simulink model "TST_CoETM_ClgDem"  (R2016b)
settings: Solver=FixedStepDiscrete  StartTime=0.0  StopTime=simTime  FixedStep=sampleTime  RelTol=1e-3
values from neighbouring files (symbols this model uses):
  testCase = 1    [initTST_CoETM_ClgDem_001.m]    (also in initTST_CoETM_ClgDem_002.m = 2)
libraries: simulink x7, UnitTest_Lib x4
settings Model: Creator=xinchangran  LastModifiedBy=xinchangran
settings DebuggingCC: SignalRangeChecking=error

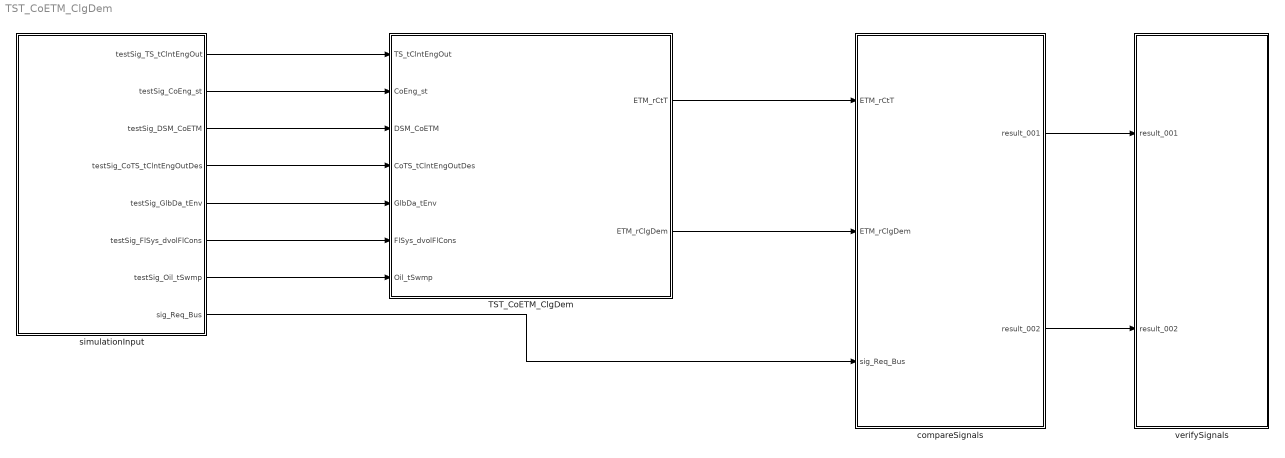
== system TST_CoETM_ClgDem ==
  TST_CoETM_ClgDem : Subsystem
  compareSignals : Subsystem
  simulationInput : Subsystem
  verifySignals : Subsystem
  wires:
  simulationInput/1(testSig_TS_tClntEngOut) -> TST_CoETM_ClgDem/1(TS_tClntEngOut)
  simulationInput/2(testSig_CoEng_st) -> TST_CoETM_ClgDem/2(CoEng_st)
  simulationInput/3(testSig_DSM_CoETM) -> TST_CoETM_ClgDem/3(DSM_CoETM)
  simulationInput/4(testSig_CoTS_tClntEngOutDes) -> TST_CoETM_ClgDem/4(CoTS_tClntEngOutDes)
  simulationInput/5(testSig_GlbDa_tEnv) -> TST_CoETM_ClgDem/5(GlbDa_tEnv)
  simulationInput/6(testSig_FlSys_dvolFlCons) -> TST_CoETM_ClgDem/6(FlSys_dvolFlCons)
  simulationInput/7(testSig_Oil_tSwmp) -> TST_CoETM_ClgDem/7(Oil_tSwmp)
  TST_CoETM_ClgDem/1(ETM_rCtT) -> compareSignals/1(ETM_rCtT)
  TST_CoETM_ClgDem/2(ETM_rClgDem) -> compareSignals/2(ETM_rClgDem)
  simulationInput/8(sig_Req_Bus) -> compareSignals/3(sig_Req_Bus)
  compareSignals/1(result_001) -> verifySignals/1(result_001)
  compareSignals/2(result_002) -> verifySignals/2(result_002)

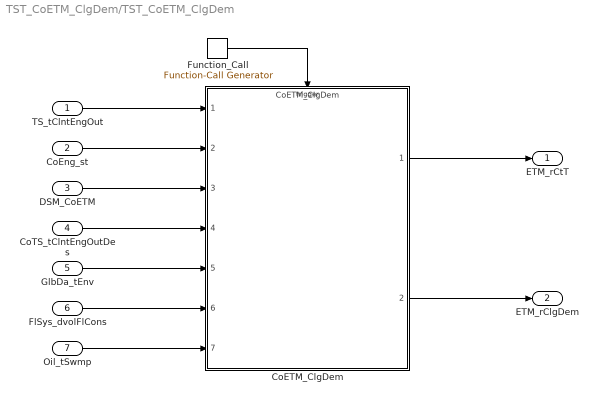
== system TST_CoETM_ClgDem/TST_CoETM_ClgDem ==
  TS_tClntEngOut : Inport
  CoEng_st : Inport  Port=2
  DSM_CoETM : Inport  Port=3
  CoTS_tClntEngOutDes : Inport  Port=4
  GlbDa_tEnv : Inport  Port=5
  FlSys_dvolFlCons : Inport  Port=6
  Oil_tSwmp : Inport  Port=7
  CoETM_ClgDem : ModelReference  ModelNameDialog=CoETM_ClgDem  SimulationMode=Normal  ModelReferenceVersion=1.155  TriggerPortName=function  TriggerPortTriggerType=function-call  TriggerPortStatesWhenEnabling=held
  Function_Call : simulink/Ports & Subsystems/Function-Call Generator  sample_time=sampleTime  numberOfIterations=1
  ETM_rCtT : Outport
  ETM_rClgDem : Outport  Port=2
  wires:
  Function_Call/1 -> CoETM_ClgDem/Trigger
  TS_tClntEngOut/1 -> CoETM_ClgDem/1
  CoEng_st/1 -> CoETM_ClgDem/2
  DSM_CoETM/1 -> CoETM_ClgDem/3
  CoTS_tClntEngOutDes/1 -> CoETM_ClgDem/4
  GlbDa_tEnv/1 -> CoETM_ClgDem/5
  FlSys_dvolFlCons/1 -> CoETM_ClgDem/6
  Oil_tSwmp/1 -> CoETM_ClgDem/7
  CoETM_ClgDem/1 -> ETM_rCtT/1
  CoETM_ClgDem/2 -> ETM_rClgDem/1

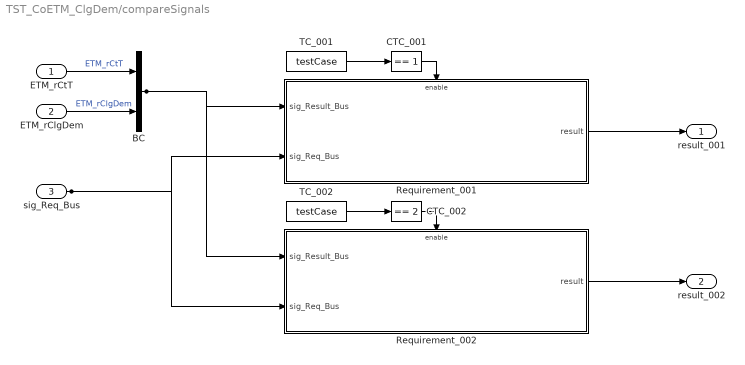
== system TST_CoETM_ClgDem/compareSignals ==
  ETM_rCtT : Inport
  ETM_rClgDem : Inport  Port=2
  sig_Req_Bus : Inport  Port=3
  BC : BusCreator  Inputs=2
  CTC_001 : simulink/Logic and Bit Operations/Compare To Constant  relop===  const=1  OutDataTypeStr=boolean
  CTC_002 : simulink/Logic and Bit Operations/Compare To Constant  relop===  const=2  OutDataTypeStr=boolean
  Requirement_001 : Subsystem
  Requirement_002 : Subsystem
  TC_001 : Constant  Value=testCase
  TC_002 : Constant  Value=testCase
  result_001 : Outport
  result_002 : Outport  Port=2
  wires:
  ETM_rCtT/1 -> BC/1  "ETM_rCtT"
  ETM_rClgDem/1 -> BC/2  "ETM_rClgDem"
  TC_001/1 -> CTC_001/1
  CTC_001/1 -> Requirement_001/Enable
  sig_Req_Bus/1 -> Requirement_001/2(sig_Req_Bus), Requirement_002/2(sig_Req_Bus)
  BC/1 -> Requirement_001/1(sig_Result_Bus), Requirement_002/1(sig_Result_Bus)
  Requirement_001/1(result) -> result_001/1
  TC_002/1 -> CTC_002/1
  CTC_002/1 -> Requirement_002/Enable
  Requirement_002/1(result) -> result_002/1

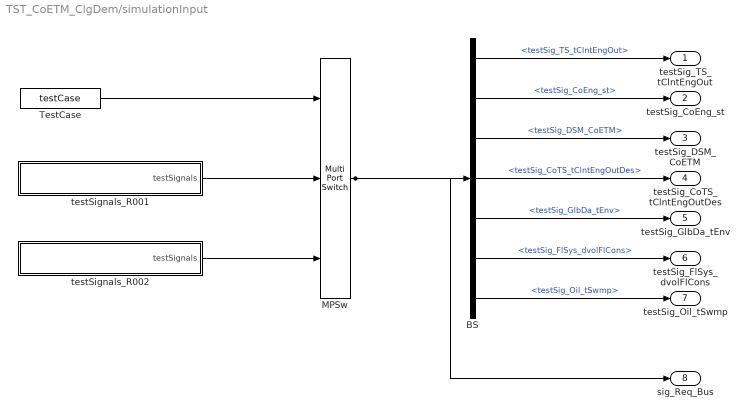
== system TST_CoETM_ClgDem/simulationInput ==
  BS : BusSelector  OutputSignals=testSig_TS_tClntEngOut,testSig_CoEng_st,testSig_DSM_CoETM,testSig_CoTS_tClntEngOutDes,testSig_GlbDa_tEnv,testSig_FlSys_dvolFlCons,testSig_Oil_tSwmp
  MPSw : MultiPortSwitch  Inputs=2  SaturateOnIntegerOverflow=on  InputSameDT=on
  TestCase : Constant  Value=testCase
  testSignals_R001 : Subsystem
  testSignals_R002 : Subsystem
  testSig_TS_tClntEngOut : Outport
  testSig_CoEng_st : Outport  Port=2
  testSig_DSM_CoETM : Outport  Port=3
  testSig_CoTS_tClntEngOutDes : Outport  Port=4
  testSig_GlbDa_tEnv : Outport  Port=5
  testSig_FlSys_dvolFlCons : Outport  Port=6
  testSig_Oil_tSwmp : Outport  Port=7
  sig_Req_Bus : Outport  Port=8
  wires:
  BS/1 -> testSig_TS_tClntEngOut/1  "<testSig_TS_tClntEngOut>"
  BS/2 -> testSig_CoEng_st/1  "<testSig_CoEng_st>"
  BS/3 -> testSig_DSM_CoETM/1  "<testSig_DSM_CoETM>"
  BS/4 -> testSig_CoTS_tClntEngOutDes/1  "<testSig_CoTS_tClntEngOutDes>"
  BS/5 -> testSig_GlbDa_tEnv/1  "<testSig_GlbDa_tEnv>"
  BS/6 -> testSig_FlSys_dvolFlCons/1  "<testSig_FlSys_dvolFlCons>"
  BS/7 -> testSig_Oil_tSwmp/1  "<testSig_Oil_tSwmp>"
  MPSw/1 -> BS/1, sig_Req_Bus/1
  TestCase/1 -> MPSw/1
  testSignals_R001/1(testSignals) -> MPSw/2
  testSignals_R002/1(testSignals) -> MPSw/3

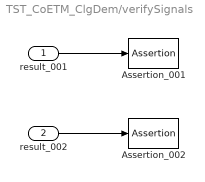
== system TST_CoETM_ClgDem/verifySignals ==
  result_001 : Inport
  result_002 : Inport  Port=2
  Assertion_001 : Assertion  Enabled=off
  Assertion_002 : Assertion  Enabled=off
  wires:
  result_001/1 -> Assertion_001/1
  result_002/1 -> Assertion_002/1

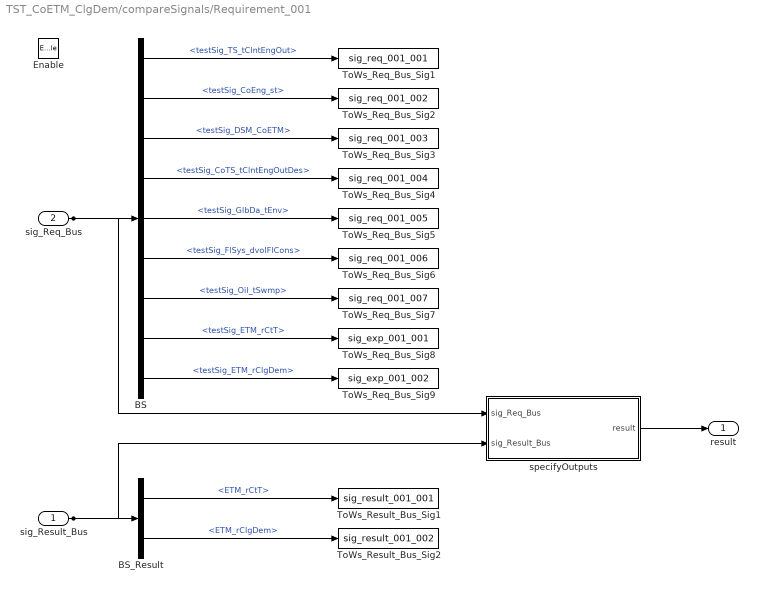
== system TST_CoETM_ClgDem/compareSignals/Requirement_001 ==
  sig_Result_Bus : Inport
  sig_Req_Bus : Inport  Port=2
  Enable : EnablePort
  BS : BusSelector  OutputSignals=testSig_TS_tClntEngOut,testSig_CoEng_st,testSig_DSM_CoETM,testSig_CoTS_tClntEngOutDes,testSig_GlbDa_tEnv,testSig_FlSys_dvolFlCons,testSig_Oil_tSwmp,testSig_ETM_rCtT,testSig_ETM_rClgDem
  BS_Result : BusSelector  OutputSignals=ETM_rCtT,ETM_rClgDem
  ToWs_Req_Bus_Sig1 : ToWorkspace  VariableName=sig_req_001_001  SaveFormat=Structure With Time
  ToWs_Req_Bus_Sig2 : ToWorkspace  VariableName=sig_req_001_002  SaveFormat=Structure With Time
  ToWs_Req_Bus_Sig3 : ToWorkspace  VariableName=sig_req_001_003  SaveFormat=Structure With Time
  ToWs_Req_Bus_Sig4 : ToWorkspace  VariableName=sig_req_001_004  SaveFormat=Structure With Time
  ToWs_Req_Bus_Sig5 : ToWorkspace  VariableName=sig_req_001_005  SaveFormat=Structure With Time
  ToWs_Req_Bus_Sig6 : ToWorkspace  VariableName=sig_req_001_006  SaveFormat=Structure With Time
  ToWs_Req_Bus_Sig7 : ToWorkspace  VariableName=sig_req_001_007  SaveFormat=Structure With Time
  ToWs_Req_Bus_Sig8 : ToWorkspace  VariableName=sig_exp_001_001  SaveFormat=Structure With Time
  ToWs_Req_Bus_Sig9 : ToWorkspace  VariableName=sig_exp_001_002  SaveFormat=Structure With Time
  ToWs_Result_Bus_Sig1 : ToWorkspace  VariableName=sig_result_001_001  SaveFormat=Structure With Time
  ToWs_Result_Bus_Sig2 : ToWorkspace  VariableName=sig_result_001_002  SaveFormat=Structure With Time
  specifyOutputs : Subsystem
  result : Outport
  wires:
  sig_Req_Bus/1 -> BS/1, specifyOutputs/1(sig_Req_Bus)
  BS/1 -> ToWs_Req_Bus_Sig1/1  "<testSig_TS_tClntEngOut>"
  BS/2 -> ToWs_Req_Bus_Sig2/1  "<testSig_CoEng_st>"
  BS/3 -> ToWs_Req_Bus_Sig3/1  "<testSig_DSM_CoETM>"
  BS/4 -> ToWs_Req_Bus_Sig4/1  "<testSig_CoTS_tClntEngOutDes>"
  BS/5 -> ToWs_Req_Bus_Sig5/1  "<testSig_GlbDa_tEnv>"
  BS/6 -> ToWs_Req_Bus_Sig6/1  "<testSig_FlSys_dvolFlCons>"
  BS/7 -> ToWs_Req_Bus_Sig7/1  "<testSig_Oil_tSwmp>"
  BS/8 -> ToWs_Req_Bus_Sig8/1  "<testSig_ETM_rCtT>"
  BS/9 -> ToWs_Req_Bus_Sig9/1  "<testSig_ETM_rClgDem>"
  sig_Result_Bus/1 -> BS_Result/1, specifyOutputs/2(sig_Result_Bus)
  BS_Result/1 -> ToWs_Result_Bus_Sig1/1  "<ETM_rCtT>"
  BS_Result/2 -> ToWs_Result_Bus_Sig2/1  "<ETM_rClgDem>"
  specifyOutputs/1(result) -> result/1

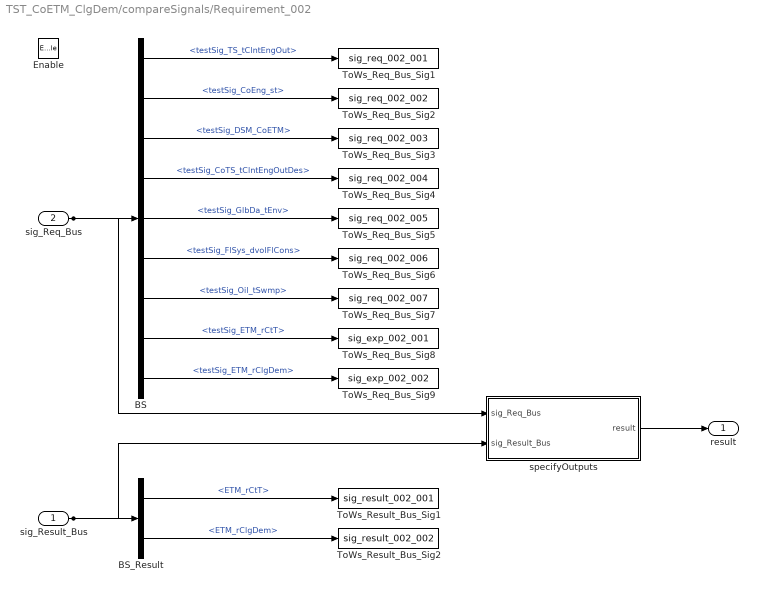
== system TST_CoETM_ClgDem/compareSignals/Requirement_002 ==
  sig_Result_Bus : Inport
  sig_Req_Bus : Inport  Port=2
  Enable : EnablePort
  BS : BusSelector  OutputSignals=testSig_TS_tClntEngOut,testSig_CoEng_st,testSig_DSM_CoETM,testSig_CoTS_tClntEngOutDes,testSig_GlbDa_tEnv,testSig_FlSys_dvolFlCons,testSig_Oil_tSwmp,testSig_ETM_rCtT,testSig_ETM_rClgDem
  BS_Result : BusSelector  OutputSignals=ETM_rCtT,ETM_rClgDem
  ToWs_Req_Bus_Sig1 : ToWorkspace  VariableName=sig_req_002_001  SaveFormat=Structure With Time
  ToWs_Req_Bus_Sig2 : ToWorkspace  VariableName=sig_req_002_002  SaveFormat=Structure With Time
  ToWs_Req_Bus_Sig3 : ToWorkspace  VariableName=sig_req_002_003  SaveFormat=Structure With Time
  ToWs_Req_Bus_Sig4 : ToWorkspace  VariableName=sig_req_002_004  SaveFormat=Structure With Time
  ToWs_Req_Bus_Sig5 : ToWorkspace  VariableName=sig_req_002_005  SaveFormat=Structure With Time
  ToWs_Req_Bus_Sig6 : ToWorkspace  VariableName=sig_req_002_006  SaveFormat=Structure With Time
  ToWs_Req_Bus_Sig7 : ToWorkspace  VariableName=sig_req_002_007  SaveFormat=Structure With Time
  ToWs_Req_Bus_Sig8 : ToWorkspace  VariableName=sig_exp_002_001  SaveFormat=Structure With Time
  ToWs_Req_Bus_Sig9 : ToWorkspace  VariableName=sig_exp_002_002  SaveFormat=Structure With Time
  ToWs_Result_Bus_Sig1 : ToWorkspace  VariableName=sig_result_002_001  SaveFormat=Structure With Time
  ToWs_Result_Bus_Sig2 : ToWorkspace  VariableName=sig_result_002_002  SaveFormat=Structure With Time
  specifyOutputs : Subsystem
  result : Outport
  wires:
  sig_Req_Bus/1 -> BS/1, specifyOutputs/1(sig_Req_Bus)
  BS/1 -> ToWs_Req_Bus_Sig1/1  "<testSig_TS_tClntEngOut>"
  BS/2 -> ToWs_Req_Bus_Sig2/1  "<testSig_CoEng_st>"
  BS/3 -> ToWs_Req_Bus_Sig3/1  "<testSig_DSM_CoETM>"
  BS/4 -> ToWs_Req_Bus_Sig4/1  "<testSig_CoTS_tClntEngOutDes>"
  BS/5 -> ToWs_Req_Bus_Sig5/1  "<testSig_GlbDa_tEnv>"
  BS/6 -> ToWs_Req_Bus_Sig6/1  "<testSig_FlSys_dvolFlCons>"
  BS/7 -> ToWs_Req_Bus_Sig7/1  "<testSig_Oil_tSwmp>"
  BS/8 -> ToWs_Req_Bus_Sig8/1  "<testSig_ETM_rCtT>"
  BS/9 -> ToWs_Req_Bus_Sig9/1  "<testSig_ETM_rClgDem>"
  sig_Result_Bus/1 -> BS_Result/1, specifyOutputs/2(sig_Result_Bus)
  BS_Result/1 -> ToWs_Result_Bus_Sig1/1  "<ETM_rCtT>"
  BS_Result/2 -> ToWs_Result_Bus_Sig2/1  "<ETM_rClgDem>"
  specifyOutputs/1(result) -> result/1

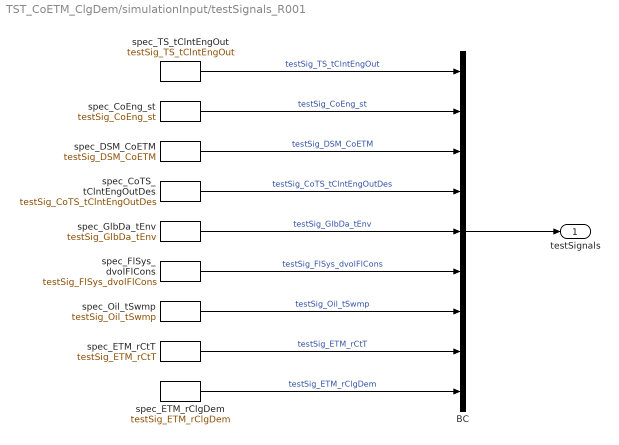
== system TST_CoETM_ClgDem/simulationInput/testSignals_R001 ==
  BC : BusCreator  Inputs=9
  spec_CoEng_st : FromWorkspace  VariableName=testSig_CoEng_st  Interpolate=off  OutputAfterFinalValue=Holding final value
  spec_CoTS_tClntEngOutDes : FromWorkspace  VariableName=testSig_CoTS_tClntEngOutDes  Interpolate=off  OutputAfterFinalValue=Holding final value
  spec_DSM_CoETM : FromWorkspace  VariableName=testSig_DSM_CoETM  Interpolate=off  OutputAfterFinalValue=Holding final value
  spec_ETM_rClgDem : FromWorkspace  VariableName=testSig_ETM_rClgDem  Interpolate=off  OutputAfterFinalValue=Holding final value
  spec_ETM_rCtT : FromWorkspace  VariableName=testSig_ETM_rCtT  Interpolate=off  OutputAfterFinalValue=Holding final value
  spec_FlSys_dvolFlCons : FromWorkspace  VariableName=testSig_FlSys_dvolFlCons  Interpolate=off  OutputAfterFinalValue=Holding final value
  spec_GlbDa_tEnv : FromWorkspace  VariableName=testSig_GlbDa_tEnv  Interpolate=off  OutputAfterFinalValue=Holding final value
  spec_Oil_tSwmp : FromWorkspace  VariableName=testSig_Oil_tSwmp  Interpolate=off  OutputAfterFinalValue=Holding final value
  spec_TS_tClntEngOut : FromWorkspace  VariableName=testSig_TS_tClntEngOut  Interpolate=off  OutputAfterFinalValue=Holding final value
  testSignals : Outport
  wires:
  BC/1 -> testSignals/1
  spec_TS_tClntEngOut/1 -> BC/1  "testSig_TS_tClntEngOut"
  spec_CoEng_st/1 -> BC/2  "testSig_CoEng_st"
  spec_DSM_CoETM/1 -> BC/3  "testSig_DSM_CoETM"
  spec_CoTS_tClntEngOutDes/1 -> BC/4  "testSig_CoTS_tClntEngOutDes"
  spec_GlbDa_tEnv/1 -> BC/5  "testSig_GlbDa_tEnv"
  spec_FlSys_dvolFlCons/1 -> BC/6  "testSig_FlSys_dvolFlCons"
  spec_Oil_tSwmp/1 -> BC/7  "testSig_Oil_tSwmp"
  spec_ETM_rCtT/1 -> BC/8  "testSig_ETM_rCtT"
  spec_ETM_rClgDem/1 -> BC/9  "testSig_ETM_rClgDem"

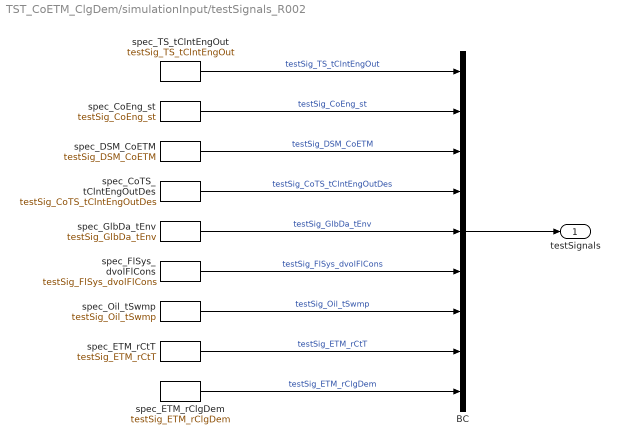
== system TST_CoETM_ClgDem/simulationInput/testSignals_R002 ==
  BC : BusCreator  Inputs=9
  spec_CoEng_st : FromWorkspace  VariableName=testSig_CoEng_st  Interpolate=off  OutputAfterFinalValue=Holding final value
  spec_CoTS_tClntEngOutDes : FromWorkspace  VariableName=testSig_CoTS_tClntEngOutDes  Interpolate=off  OutputAfterFinalValue=Holding final value
  spec_DSM_CoETM : FromWorkspace  VariableName=testSig_DSM_CoETM  Interpolate=off  OutputAfterFinalValue=Holding final value
  spec_ETM_rClgDem : FromWorkspace  VariableName=testSig_ETM_rClgDem  Interpolate=off  OutputAfterFinalValue=Holding final value
  spec_ETM_rCtT : FromWorkspace  VariableName=testSig_ETM_rCtT  Interpolate=off  OutputAfterFinalValue=Holding final value
  spec_FlSys_dvolFlCons : FromWorkspace  VariableName=testSig_FlSys_dvolFlCons  Interpolate=off  OutputAfterFinalValue=Holding final value
  spec_GlbDa_tEnv : FromWorkspace  VariableName=testSig_GlbDa_tEnv  Interpolate=off  OutputAfterFinalValue=Holding final value
  spec_Oil_tSwmp : FromWorkspace  VariableName=testSig_Oil_tSwmp  Interpolate=off  OutputAfterFinalValue=Holding final value
  spec_TS_tClntEngOut : FromWorkspace  VariableName=testSig_TS_tClntEngOut  Interpolate=off  OutputAfterFinalValue=Holding final value
  testSignals : Outport
  wires:
  BC/1 -> testSignals/1
  spec_TS_tClntEngOut/1 -> BC/1  "testSig_TS_tClntEngOut"
  spec_CoEng_st/1 -> BC/2  "testSig_CoEng_st"
  spec_DSM_CoETM/1 -> BC/3  "testSig_DSM_CoETM"
  spec_CoTS_tClntEngOutDes/1 -> BC/4  "testSig_CoTS_tClntEngOutDes"
  spec_GlbDa_tEnv/1 -> BC/5  "testSig_GlbDa_tEnv"
  spec_FlSys_dvolFlCons/1 -> BC/6  "testSig_FlSys_dvolFlCons"
  spec_Oil_tSwmp/1 -> BC/7  "testSig_Oil_tSwmp"
  spec_ETM_rCtT/1 -> BC/8  "testSig_ETM_rCtT"
  spec_ETM_rClgDem/1 -> BC/9  "testSig_ETM_rClgDem"

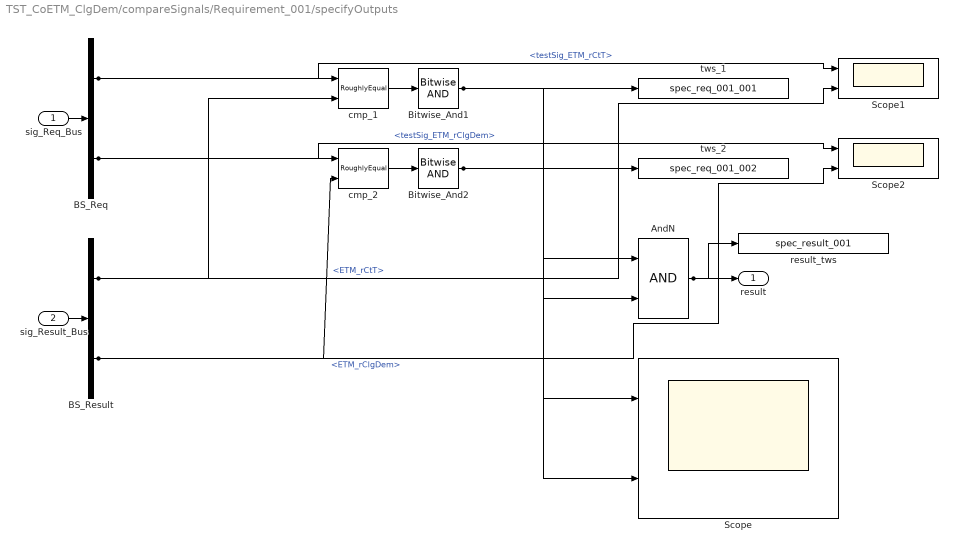
== system TST_CoETM_ClgDem/compareSignals/Requirement_001/specifyOutputs ==
  sig_Req_Bus : Inport
  sig_Result_Bus : Inport  Port=2
  AndN : Logic
  BS_Req : BusSelector  OutputSignals=testSig_ETM_rCtT,testSig_ETM_rClgDem
  BS_Result : BusSelector  OutputSignals=ETM_rCtT,ETM_rClgDem
  Bitwise_And1 : simulink/Logic and Bit Operations/Bitwise Operator  logicop=AND  UseBitMask=off  BitMask=bin2dec('11011001')  BitMaskRealWorld=Stored Integer
  Bitwise_And2 : simulink/Logic and Bit Operations/Bitwise Operator  logicop=AND  UseBitMask=off  BitMask=bin2dec('11011001')  BitMaskRealWorld=Stored Integer
  Scope : Scope  NumInputPorts=2
  Scope1 : Scope  NumInputPorts=2
  Scope2 : Scope  NumInputPorts=2
  cmp_1 : UnitTest_Lib/RoughlyEqual  slope=0.1
  cmp_2 : UnitTest_Lib/RoughlyEqual  slope=0.1
  result_tws : ToWorkspace  VariableName=spec_result_001
  tws_1 : ToWorkspace  VariableName=spec_req_001_001
  tws_2 : ToWorkspace  VariableName=spec_req_001_002
  result : Outport
  wires:
  sig_Req_Bus/1 -> BS_Req/1
  sig_Result_Bus/1 -> BS_Result/1
  AndN/1 -> result/1, result_tws/1
  BS_Req/1 -> cmp_1/1, Scope1/1  "<testSig_ETM_rCtT>"
  BS_Result/1 -> cmp_1/2, Scope1/2  "<ETM_rCtT>"
  cmp_1/1 -> Bitwise_And1/1
  Bitwise_And1/1 -> tws_1/1, AndN/1, Scope/1
  BS_Req/2 -> cmp_2/1, Scope2/1  "<testSig_ETM_rClgDem>"
  BS_Result/2 -> cmp_2/2, Scope2/2  "<ETM_rClgDem>"
  cmp_2/1 -> Bitwise_And2/1
  Bitwise_And2/1 -> tws_2/1, AndN/2, Scope/2

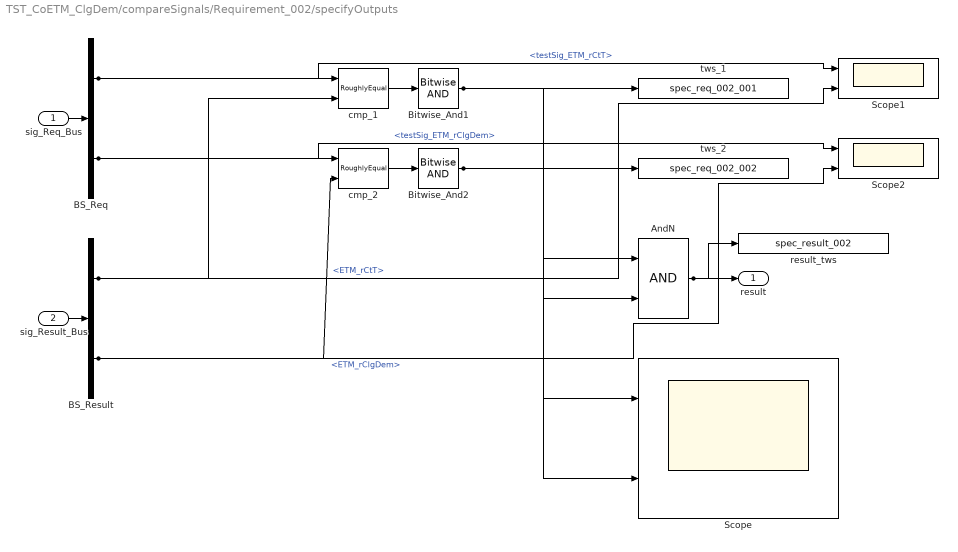
== system TST_CoETM_ClgDem/compareSignals/Requirement_002/specifyOutputs ==
  sig_Req_Bus : Inport
  sig_Result_Bus : Inport  Port=2
  AndN : Logic
  BS_Req : BusSelector  OutputSignals=testSig_ETM_rCtT,testSig_ETM_rClgDem
  BS_Result : BusSelector  OutputSignals=ETM_rCtT,ETM_rClgDem
  Bitwise_And1 : simulink/Logic and Bit Operations/Bitwise Operator  logicop=AND  UseBitMask=off  BitMask=bin2dec('11011001')  BitMaskRealWorld=Stored Integer
  Bitwise_And2 : simulink/Logic and Bit Operations/Bitwise Operator  logicop=AND  UseBitMask=off  BitMask=bin2dec('11011001')  BitMaskRealWorld=Stored Integer
  Scope : Scope  NumInputPorts=2
  Scope1 : Scope  NumInputPorts=2
  Scope2 : Scope  NumInputPorts=2
  cmp_1 : UnitTest_Lib/RoughlyEqual  slope=0.1
  cmp_2 : UnitTest_Lib/RoughlyEqual  slope=0.1
  result_tws : ToWorkspace  VariableName=spec_result_002
  tws_1 : ToWorkspace  VariableName=spec_req_002_001
  tws_2 : ToWorkspace  VariableName=spec_req_002_002
  result : Outport
  wires:
  sig_Req_Bus/1 -> BS_Req/1
  sig_Result_Bus/1 -> BS_Result/1
  AndN/1 -> result/1, result_tws/1
  BS_Req/1 -> cmp_1/1, Scope1/1  "<testSig_ETM_rCtT>"
  BS_Result/1 -> cmp_1/2, Scope1/2  "<ETM_rCtT>"
  cmp_1/1 -> Bitwise_And1/1
  Bitwise_And1/1 -> tws_1/1, AndN/1, Scope/1
  BS_Req/2 -> cmp_2/1, Scope2/1  "<testSig_ETM_rClgDem>"
  BS_Result/2 -> cmp_2/2, Scope2/2  "<ETM_rClgDem>"
  cmp_2/1 -> Bitwise_And2/1
  Bitwise_And2/1 -> tws_2/1, AndN/2, Scope/2
